simulink model "control_system"  (R2021b)
settings: Solver=VariableStepAuto  StartTime=0.0  StopTime=5  RelTol=1e-3
undefined symbols (not defined in the file or in its folder): theta_0
settings Model: Creator=jcron  LastModifiedBy=jcron

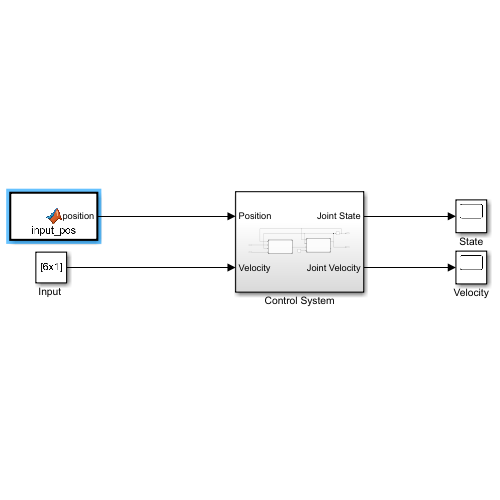
[thumbnail: Simulink's stored preview of the top-level diagram]
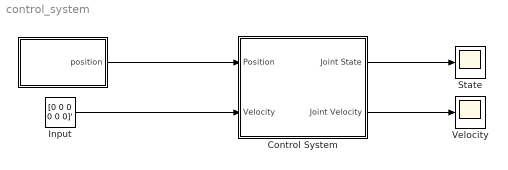
== system control_system ==
  " " : MATLAB Function  TreatAsAtomicUnit=on
  Control System : Subsystem
  "Input " : Constant  Value=[0 0 0 0 0 0]'
  State : Scope
  Velocity : Scope
  wires:
  "Input "/1 -> Control System/2(Velocity)
  " "/1(position) -> Control System/1(Position)
  Control System/1(Joint State) -> State/1
  Control System/2(Joint Velocity) -> Velocity/1

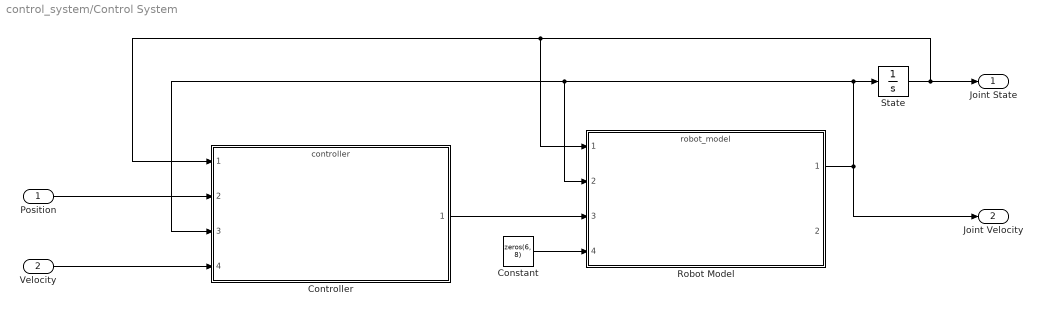
== system control_system/Control System ==
  Position : Inport  PortDimensions=[4 4]
  Velocity : Inport  Port=2  PortDimensions=[6 1]
  Constant : Constant  Value=zeros(6, 8)
  Controller : ModelReference  ModelNameDialog=controller.slx  SimulationMode=Normal  ModelReferenceVersion=1.51
  Robot Model : ModelReference  ModelNameDialog=robot_model.slx  SimulationMode=Normal  ModelReferenceVersion=1.6
  State : Integrator  InitialCondition=theta_0
  Joint State : Outport
  Joint Velocity : Outport  Port=2
  wires:
  State/1 -> Joint State/1, Controller/1, Robot Model/1
  Robot Model/1 -> Robot Model/2, Controller/3, State/1, Joint Velocity/1
  Velocity/1 -> Controller/4
  Position/1 -> Controller/2
  Constant/1 -> Robot Model/4
  Controller/1 -> Robot Model/3

== matlab function control_system/  ==
  data: position output
function position = input_pos()
position = zeros(4, 4);
% expm(pi * skew3([1 0 0]'));
position(1:3, 1:3) = [
    0 0 -1;
    0 -1 0;
    -1 0 0
];
position(1:3, 4) = [-15 0 -10]';
position(4, 4) = 1;
